simulink model "completo"  (R2022a)
settings: Solver=ode5  StartTime=0.0  StopTime=15  FixedStep=0.0001  RelTol=1e-3
InitFcn:
  | params_completo
values from neighbouring files (symbols this model uses):
  a = -1  /tau    (= -1000)    [params_completo.m]
  A_h = 0.40648    [params_completo.m]
  a_sat = (pi)/(2*(M_ij - L_ij))    (= 0.0314159265359)    [params_completo.m]
  alpha = 80    [params_completo.m]
  b = 1/tau    (= 1000)    [params_completo.m]
  beta1 = 0.0032    [params_completo.m]
  beta2 = 0.0035    [params_completo.m]
  beta3 = -0.0010    (= -0.001)    [params_completo.m]
  beta4 = -0.0003    [params_completo.m]
  beta5 = -0.0002    [params_completo.m]
  beta6 = 0.0004    [params_completo.m]
  freq = 2*pi/10    (= 0.628318530718)    [params_completo.m]
  k = 1.0773    [params_completo.m]
  k1 = 20    [params_completo.m]
  k1_o = 500    [params_completo.m]
  k2_o = 200    [params_completo.m]
  kx1 = 800    [params_completo.m]
  kx2 = 200    [params_completo.m]
  L_ij = 450    [params_completo.m]
  mu1 = 0.2    [params_completo.m]
  mu2 = 1.2    [params_completo.m]
  Phi_sum_abs = abs(beta1) + abs(beta2) + abs(beta3) +                abs(beta4) + abs(beta5) + abs(beta6)    [params_completo.m]
  Phi_sum_abs_ESTIMATED = Phi_sum_abs + 0.1 * Phi_sum_abs    [params_completo.m]
  q = 1    [params_completo.m]
settings Model: Creator=gerar  LastModifiedBy=CIO
settings SolverCC: AlgebraicLoopSolver=TrustRegion
settings DebuggingCC: UnconnectedInputMsg=warning  UnconnectedOutputMsg=warning  UnconnectedLineMsg=warning  SFMachineParentedDataDiag=warning
settings SFSimCC: CustomCodeUndefinedFunction=UseInterfaceOnly
settings RTWCC: DLArmComputeVersion=19.05

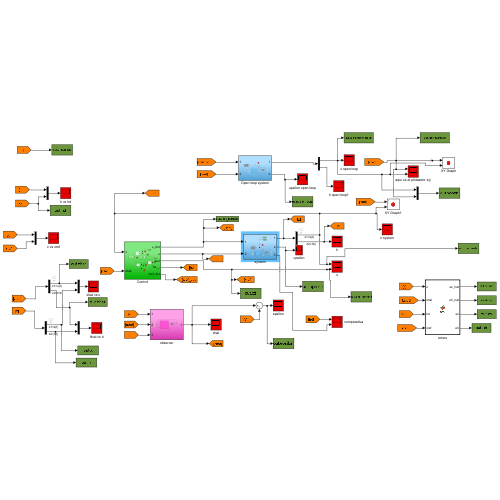
[thumbnail: Simulink's stored preview of the top-level diagram]
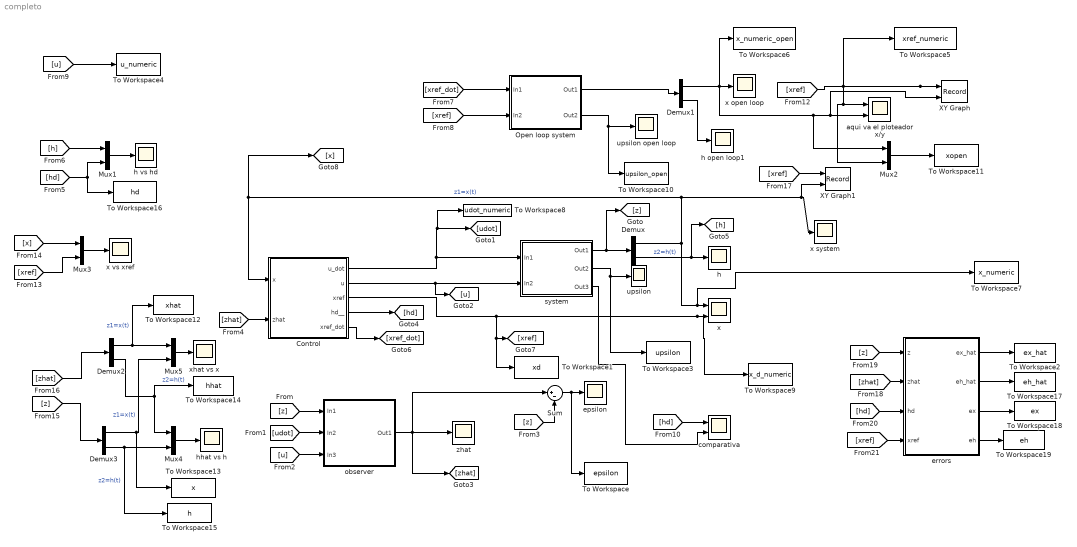
== system completo ==
  Control : Subsystem
  Demux{,1..3} (4 alike) : Demux  Outputs=2
  Mux{1..5} (5 alike) : Mux  Inputs=2
  Open loop system : Subsystem
  Sum : Sum  Inputs=|+-
  To Workspace : ToWorkspace  VariableName=epsilon  SaveFormat=Timeseries  SampleTime=-1
  To Workspace1 : ToWorkspace  VariableName=xd  SaveFormat=Timeseries  SampleTime=-1
  To Workspace10 : ToWorkspace  VariableName=upsilon_open  SaveFormat=Structure  SampleTime=-1
  To Workspace11 : ToWorkspace  VariableName=xopen  SaveFormat=Timeseries  SampleTime=-1
  To Workspace12 : ToWorkspace  VariableName=xhat  SaveFormat=Timeseries  SampleTime=-1
  To Workspace13 : ToWorkspace  VariableName=x  SaveFormat=Timeseries  SampleTime=-1
  To Workspace14 : ToWorkspace  VariableName=hhat  SaveFormat=Timeseries  SampleTime=-1
  To Workspace15 : ToWorkspace  VariableName=h  SaveFormat=Timeseries  SampleTime=-1
  To Workspace16 : ToWorkspace  VariableName=hd  SaveFormat=Timeseries  SampleTime=-1
  To Workspace17 : ToWorkspace  VariableName=eh_hat  SaveFormat=Timeseries  SampleTime=-1
  To Workspace18 : ToWorkspace  VariableName=ex  SaveFormat=Timeseries  SampleTime=-1
  To Workspace19 : ToWorkspace  VariableName=eh  SaveFormat=Timeseries  SampleTime=-1
  To Workspace2 : ToWorkspace  VariableName=ex_hat  SaveFormat=Timeseries  SampleTime=-1
  To Workspace3 : ToWorkspace  VariableName=upsilon  SaveFormat=Structure  SampleTime=-1
  To Workspace4 : ToWorkspace  VariableName=u_numeric  SaveFormat=Structure  SampleTime=-1
  To Workspace5 : ToWorkspace  VariableName=xref_numeric  SaveFormat=Structure  SampleTime=-1
  To Workspace6 : ToWorkspace  VariableName=x_numeric_open  SaveFormat=Structure  SampleTime=-1
  To Workspace7 : ToWorkspace  VariableName=x_numeric  SaveFormat=Structure  SampleTime=-1
  To Workspace8 : ToWorkspace  VariableName=udot_numeric  SaveFormat=Structure  SampleTime=-1
  To Workspace9 : ToWorkspace  VariableName=x_d_numeric  SaveFormat=Structure  SampleTime=-1
  XY Graph : Record  FileSettingsInternal="{\"entries\":[{\"content\":{\"excelSettings\":{\"content\":{},\"type\":\"Streamout.ExcelSettings\"}},\"type\":\"Streamout.FileSettingStorage\",\"uuid\":\"58948ec6-d345-4ba4-a5f9-32bad8470a1a\"}],\"packageUris\":[\"http://schema.mathworks.com/mf0/streamout_blocks/R2020a\"],\"version\":\"1.0\"}"  Layout=[1 1]  SignalsInternal="{\"entries\":[{\"content\":{\"signals\":[{\"content\":{\"blockPath\":[\"completo/XY Graph\"],\"channel\":[],\"dimensions\":[1],\"domain\":\"completo/XY Graph\",\"lineColor\":\"#a2142f\",\"plots\":[1],\"port\":1,\"sid\":[],\"signalID\":655,\"signalName\":\"From12\"},\"type\":\"RecordBlkView.Signal\",\"uuid\":\"ccf76168-5501-4964-b812-cd25957922a2\"},{\"content\":{\"blockPath\":[\"completo/XY Graph\"],\"channel\":[],\"dimensions\":[1],\"domain\":\"completo/XY Graph\",\"lineColor\":\"#139fff\",\"plots\":[1],\"port\":2,\"sid\":[],\"signalID\":658,\"signalName\":\"Demux1:1\"},\"type\":\"RecordBlkView.Signal\",\"uuid\":\"d05795eb-9c31-488d-9f29-71855a3ce2a9\"}]},\"type\":\"RecordBlkView.InputSignals\",\"uuid\":\"1ab41c32-35a5-46b4-97f6-ee8bfd3e0af7\"}],\"packageUris\":[\"http://schema.mathworks.com/mf0/streamout_blocks/R2020a\"],\"version\":\"1.0\"}"  VisualizationBindings="{\"xyplotplugin\":{\"info\":[{\"series\":[{\"bindingParametersList\":[{\"parameter\":\"X-Axis\",\"signalID\":655,\"signalName\":\"From12\"},{\"parameter\":\"Y-Axis\",\"signalID\":658,\"signalName\":\"Demux1:1\"}],\"seriesID\":39720}],\"subplotID\":1}]}}"  CompatibilityTag=XY
  XY Graph1 : Record  FileSettingsInternal="{\"entries\":[{\"content\":{\"excelSettings\":{\"content\":{},\"type\":\"Streamout.ExcelSettings\"}},\"type\":\"Streamout.FileSettingStorage\",\"uuid\":\"11f322b1-eef3-45be-a83d-5182385591cb\"}],\"packageUris\":[\"http://schema.mathworks.com/mf0/streamout_blocks/R2020a\"],\"version\":\"1.0\"}"  Layout=[1 1]  SignalsInternal="{\"entries\":[{\"content\":{\"signals\":[{\"content\":{\"blockPath\":[\"completo/XY Graph1\"],\"channel\":[],\"dimensions\":[1],\"domain\":\"completo/XY Graph1\",\"lineColor\":\"#a2142f\",\"plots\":[1],\"port\":1,\"sid\":[],\"signalID\":647,\"signalName\":\"From17\"},\"type\":\"RecordBlkView.Signal\",\"uuid\":\"a2b6a24d-7c32-44e8-9cda-e5b06c3ad770\"},{\"content\":{\"blockPath\":[\"completo/XY Graph1\"],\"channel\":[],\"dimensions\":[1],\"domain\":\"completo/XY Graph1\",\"lineColor\":\"#139fff\",\"plots\":[1],\"port\":2,\"sid\":[],\"signalID\":650,\"signalName\":\"z1=x(t)\"},\"type\":\"RecordBlkView.Signal\",\"uuid\":\"9a324e81-d58f-46a3-8cfa-1b0d0714c485\"}]},\"type\":\"RecordBlkView.InputSignals\",\"uuid\":\"4fdf8df6-887b-4fd8-83f4-ac5bb18b92d4\"}],\"packageUris\":[\"http://schema.mathworks.com/mf0/streamout_blocks/R2020a\"],\"version\":\"1.0\"}"  VisualizationBindings="{\"xyplotplugin\":{\"info\":[{\"series\":[{\"bindingParametersList\":[{\"parameter\":\"X-Axis\",\"signalID\":647,\"signalName\":\"From17\"},{\"parameter\":\"Y-Axis\",\"signalID\":650,\"signalName\":\"z1=x(t)\"}],\"seriesID\":20684}],\"subplotID\":1}]}}"  CompatibilityTag=XY
  aqui va el ploteador x/y : Scope  NumInputPorts=2
  comparativa : Scope  NumInputPorts=2
  epsilon : Scope
  errors : MATLAB Function  TreatAsAtomicUnit=on
  h : Scope
  h open loop1 : Scope
  h vs hd : Scope
  hhat vs h : Scope
  observer : Subsystem
  system : Subsystem
  upsilon : Scope
  upsilon open loop : Scope
  x : Scope  NumInputPorts=2
  x open loop : Scope
  x system : Scope
  x vs xref : Scope
  xhat vs x : Scope
  zhat : Scope
  wires:
  Control/1(u_dot) -> To Workspace8/1, [udot], system/1(In1)
  Control/2(u) -> system/2(In2), [u]
  Control/3(xref) -> To Workspace1/1, [xref], To Workspace9/1, x/2
  Demux/2 -> [h], h/1  "z2=h(t)"
  Demux/1 -> To Workspace7/1, x/1, XY Graph1/2, x system/1, [x], Control/1(x)  "z1=x(t)"
  system/1(Out1) -> Demux/1, [z]
  [z] -> observer/1(In1)
  observer/1(Out1) -> [zhat], Sum/1, zhat/1
  [udot] -> observer/2(In2)
  [u] -> observer/3(In3)
  [z] -> Sum/2
  Sum/1 -> To Workspace/1, epsilon/1
  [zhat] -> Control/2(zhat)
  system/2(Out2) -> To Workspace3/1, upsilon/1
  Control/4(hd__) -> [hd]
  [h] -> Mux1/1
  [hd] -> To Workspace16/1, Mux1/2
  Mux1/1 -> h vs hd/1
  Control/5(xref_dot) -> [xref_dot]
  [xref_dot] -> Open loop system/1(In1)
  [xref] -> Open loop system/2(In2)
  Open loop system/1(Out1) -> Demux1/1
  Open loop system/2(Out2) -> To Workspace10/1, upsilon open loop/1
  Demux1/2 -> h open loop1/1
  Demux1/1 -> To Workspace6/1, x open loop/1, XY Graph/2, aqui va el ploteador x/y/2, Mux2/1
  [u] -> To Workspace4/1
  system/3(Out3) -> comparativa/2
  [hd] -> comparativa/1
  [xref] -> XY Graph/1, To Workspace5/1, Mux2/2, aqui va el ploteador x/y/1
  Mux2/1 -> To Workspace11/1
  [xref] -> Mux3/2
  [x] -> Mux3/1
  Mux3/1 -> x vs xref/1
  [xref] -> XY Graph1/1
  [zhat] -> Demux2/1
  [z] -> Demux3/1
  Demux2/1 -> To Workspace12/1, Mux5/1  "z1=x(t)"
  Demux3/1 -> To Workspace13/1, Mux5/2  "z1=x(t)"
  Mux5/1 -> xhat vs x/1
  Demux2/2 -> To Workspace14/1, Mux4/1  "z2=h(t)"
  Demux3/2 -> To Workspace15/1, Mux4/2  "z2=h(t)"
  Mux4/1 -> hhat vs h/1
  [zhat] -> errors/2(zhat)
  [z] -> errors/1(z)
  [hd] -> errors/3(hd)
  [xref] -> errors/4(xref)
  errors/1(ex_hat) -> To Workspace2/1
  errors/2(eh_hat) -> To Workspace17/1
  errors/3(ex) -> To Workspace18/1
  errors/4(eh) -> To Workspace19/1

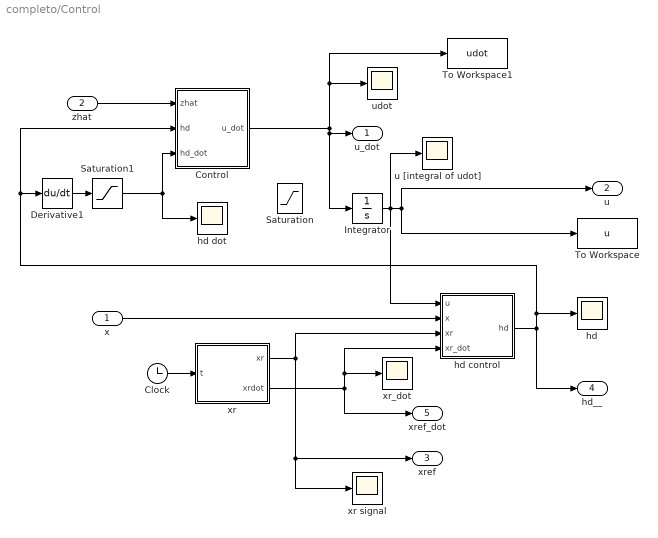
== system completo/Control ==
  x : Inport
  zhat : Inport  Port=2
  Clock : Clock
  Control : MATLAB Function  TreatAsAtomicUnit=on
  Derivative1 : Derivative
  Integrator : Integrator
  Saturation : Saturate  UpperLimit=100  LowerLimit=-100
  Saturation1 : Saturate  UpperLimit=40  LowerLimit=-40
  To Workspace : ToWorkspace  VariableName=u  SaveFormat=Timeseries  SampleTime=-1
  To Workspace1 : ToWorkspace  VariableName=udot  SaveFormat=Timeseries  SampleTime=-1
  hd : Scope
  hd control : MATLAB Function  TreatAsAtomicUnit=on
  hd dot : Scope
  u [integral of udot] : Scope
  udot : Scope
  xr : MATLAB Function  TreatAsAtomicUnit=on
  xr signal : Scope
  xr_dot : Scope
  u_dot : Outport  VectorParamsAs1DForOutWhenUnconnected=off
  u : Outport  Port=2  VectorParamsAs1DForOutWhenUnconnected=off
  xref : Outport  Port=3  VectorParamsAs1DForOutWhenUnconnected=off
  hd__ : Outport  Port=4  VectorParamsAs1DForOutWhenUnconnected=off
  xref_dot : Outport  Port=5  VectorParamsAs1DForOutWhenUnconnected=off
  wires:
  Integrator/1 -> hd control/1(u), To Workspace/1, u/1, u [integral of udot]/1
  x/1 -> hd control/2(x)
  Clock/1 -> xr/1(t)
  xr/1(xr) -> xr signal/1, xref/1, hd control/3(xr)
  zhat/1 -> Control/1(zhat)
  xr/2(xrdot) -> xref_dot/1, hd control/4(xr_dot), xr_dot/1
  Derivative1/1 -> Saturation1/1
  Saturation1/1 -> hd dot/1, Control/3(hd_dot)
  hd control/1(hd) -> hd/1, Control/2(hd), Derivative1/1, hd__/1
  Control/1(u_dot) -> Integrator/1, u_dot/1, udot/1, To Workspace1/1

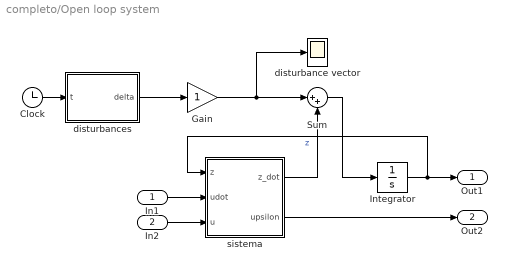
== system completo/Open loop system ==
  In1 : Inport
  In2 : Inport  Port=2
  Clock : Clock
  Gain : Gain
  Integrator : Integrator  InitialCondition=[3;-2]
  Sum : Sum  Inputs=|++
  disturbance vector : Scope
  disturbances : MATLAB Function  TreatAsAtomicUnit=on
  sistema : MATLAB Function  TreatAsAtomicUnit=on
  Out1 : Outport  VectorParamsAs1DForOutWhenUnconnected=off
  Out2 : Outport  Port=2  VectorParamsAs1DForOutWhenUnconnected=off
  wires:
  Integrator/1 -> Out1/1, sistema/1(z)  "z"
  In1/1 -> sistema/2(udot)
  In2/1 -> sistema/3(u)
  sistema/2(upsilon) -> Out2/1
  Clock/1 -> disturbances/1(t)
  sistema/1(z_dot) -> Sum/2
  disturbances/1(delta) -> Gain/1
  Sum/1 -> Integrator/1
  Gain/1 -> Sum/1, disturbance vector/1

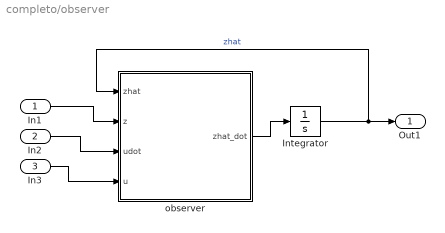
== system completo/observer ==
  In1 : Inport
  In2 : Inport  Port=2
  In3 : Inport  Port=3
  Integrator : Integrator  InitialCondition=[0;0]
  observer : MATLAB Function  TreatAsAtomicUnit=on
  Out1 : Outport  VectorParamsAs1DForOutWhenUnconnected=off
  wires:
  observer/1(zhat_dot) -> Integrator/1
  Integrator/1 -> observer/1(zhat), Out1/1  "zhat"
  In1/1 -> observer/2(z)
  In2/1 -> observer/3(udot)
  In3/1 -> observer/4(u)

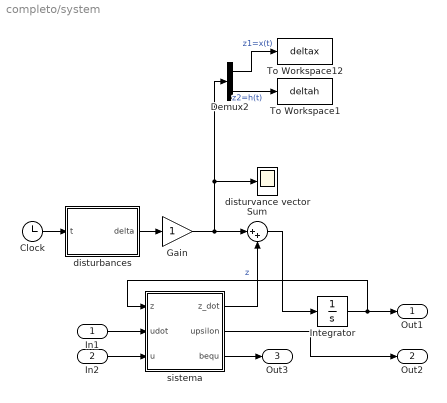
== system completo/system ==
  In1 : Inport
  In2 : Inport  Port=2
  Clock : Clock
  Demux2 : Demux  Outputs=2
  Gain : Gain
  Integrator : Integrator  InitialCondition=[3;-2]
  Sum : Sum  Inputs=|++
  To Workspace1 : ToWorkspace  VariableName=deltah  SaveFormat=Timeseries  SampleTime=-1
  To Workspace12 : ToWorkspace  VariableName=deltax  SaveFormat=Timeseries  SampleTime=-1
  disturbances : MATLAB Function  TreatAsAtomicUnit=on
  disturvance vector : Scope
  sistema : MATLAB Function  TreatAsAtomicUnit=on
  Out1 : Outport  VectorParamsAs1DForOutWhenUnconnected=off
  Out2 : Outport  Port=2  VectorParamsAs1DForOutWhenUnconnected=off
  Out3 : Outport  Port=3  VectorParamsAs1DForOutWhenUnconnected=off
  wires:
  Integrator/1 -> Out1/1, sistema/1(z)  "z"
  In1/1 -> sistema/2(udot)
  In2/1 -> sistema/3(u)
  sistema/2(upsilon) -> Out2/1
  Clock/1 -> disturbances/1(t)
  sistema/1(z_dot) -> Sum/2
  disturbances/1(delta) -> Gain/1
  Sum/1 -> Integrator/1
  sistema/3(bequ) -> Out3/1
  Gain/1 -> Demux2/1, disturvance vector/1, Sum/1
  Demux2/1 -> To Workspace12/1  "z1=x(t)"
  Demux2/2 -> To Workspace1/1  "z2=h(t)"

== matlab function completo/Open loop system/disturbances ==
  data: t input; delta output
function delta = dist(t)

delta_x = -3 - 10*cos(0.2*t+10);
delta_h = 8*sin(t); 

delta = [delta_x ; delta_h];

== matlab function completo/Open loop system/sistema ==
  data: z input; udot input; u input; z_dot output; k parameter; a parameter; b parameter; upsilon output; beta1 parameter; beta2 parameter; beta3 parameter; beta4 parameter; beta5 parameter; beta6 parameter; A_h parameter
function [z_dot, upsilon] = sys(z, udot, u, k, a, b, beta1, beta2, beta3, beta4, beta5, beta6, A_h)

    x = z(1,1);
    h = z(2,1);

    Phi = beta1*sign( udot*h ) + beta2*sign( udot*u ) + ...
          beta3*sign( u*h )    + beta4*sign( udot )   + ...
          beta5*sign( h )      + beta6*sign( u );

    %============================ System model ============================
    z_dot = [ a*x + b*k*u - b*h    ;    
            udot*( A_h - abs(h)*Phi ) ];

    upsilon = k*u - h;
    bequ = b*k*u;

== matlab function completo/errors ==
  data: z input; zhat input; hd input; ex_hat output; xref input; eh_hat output; ex output; eh output
function [ex_hat, eh_hat, ex, eh] = fcn(z, zhat, hd, xref)

x = z(1,1);
h = z(2,1);

xhat = zhat(1,1);
hhat = zhat(2,1);



%%%
ex_hat = xhat - x;
eh_hat = hhat - h;

ex = x - xref;
eh = h - hd;

== matlab function completo/Control/Control ==
  data: zhat input; hd input; hd_dot input; u_dot output; k1 parameter; A_h parameter; Phi_sum_abs parameter; Phi_sum_abs_ESTIMATED parameter
function u_dot = fcn(zhat, hd, hd_dot, k1, A_h, Phi_sum_abs, Phi_sum_abs_ESTIMATED)

eh = zhat(2,1) - hd;  %error with estimated states

%%%%%%%%%%%%%%%%%%% CO N T R O L %%%%%%%%%%%%%%%%%%%%%%%%%%%%%%%%%

u_dot = ( - k1 * sign(eh) + hd_dot )/( A_h - (Phi_sum_abs)*abs(eh + hd) ) ;

== matlab function completo/system/disturbances ==
  data: t input; delta output
function delta = dist(t)

delta_x = -3 - 10*cos(0.2*t+10);
delta_h = 8*sin(t); 

delta = [delta_x ; delta_h];

== matlab function completo/observer/observer ==
  data: zhat input; z input; udot input; u input; zhat_dot output; A_h parameter; k parameter; a parameter; b parameter; Phi_sum_abs_ESTIMATED parameter; k1_o parameter; k2_o parameter; mu1 parameter; mu2 parameter; q parameter
function zhat_dot = obs(zhat, z, udot, u, A_h, k, a, b, Phi_sum_abs_ESTIMATED, k1_o, k2_o, mu1, mu2, q)

x = z(1,1);
xhat = zhat(1,1);
hhat = zhat(2,1);


    gx = [ a*xhat + b*k*u - b*hhat                        ; %    gx = [ a*xhat + b*k*u                          ; 
          ( udot ) * ( A_h - abs(hhat)*Phi_sum_abs_ESTIMATED ) ] ;


%%%%%%%%%%%%%%%%%%%%%%%% o b s e r v e r %%%%%%%%%%%%%%%%%%%%%%%%%%%%%%%%%%
%error
e1 = xhat - x; 

%functions
phi1 = mu1*abs(e1)^(1/2)*sign(e1) + mu2 * abs(e1)^q * sign(e1)      ; 
phi2 = ( (mu1/2)*abs(e1)^(-1/2) + mu2*q*abs(e1)^(q-1) ) * ( phi1 ); 
correction_term = [- k1_o * phi1;
                   - k2_o * phi2];

zhat_dot =  gx -  correction_term;

== matlab function completo/Control/hd control ==
  data: u input; x input; xr input; xr_dot input; hd output; k parameter; a parameter; b parameter; L_ij parameter; kx1 parameter; kx2 parameter; a_sat parameter
function hd = fcn(u, x, xr, xr_dot, k, a, b, L_ij, kx1, kx2, a_sat)

ex = x - xr;

%%%%%%%%%%%%%%%%%%%%%%%% C O N T R O L  %%%%%%%%%%%%%%%%%%%%%%%%%%%

s = kx1*ex; % kx1

if s > L_ij
    sigma = tanh(a_sat*(s - L_ij))/(a_sat) + L_ij;
elseif abs(s) <= L_ij
    sigma = s;
elseif s < (-L_ij)
    sigma = tanh(a_sat*(s + L_ij))/(a_sat) - L_ij;
else
    sigma = 0;
end
    
hd = (1/b) * ( - sigma - kx2*sign(ex) + a*(ex + xr) + b*k*u - xr_dot );

== matlab function completo/Control/xr ==
  data: t input; xr output; alpha parameter; xrdot output; freq parameter
function [xr, xrdot] = fcn(t, alpha, freq)

xr = alpha*sin(freq*t);
xrdot = freq*alpha*cos(freq*t);

== matlab function completo/system/sistema ==
  data: z input; udot input; u input; z_dot output; A_h parameter; k parameter; a parameter; b parameter; upsilon output; bequ output; beta1 parameter; beta2 parameter; beta3 parameter; beta4 parameter; beta5 parameter; beta6 parameter
function [z_dot, upsilon, bequ] = sys(z, udot, u, A_h, k, a, b, beta1, beta2, beta3, beta4, beta5, beta6)

    x = z(1,1);
    h = z(2,1);

    Phi = beta1*sign( udot*h ) + beta2*sign( udot*u ) + ...
          beta3*sign( u*h )    + beta4*sign( udot )   + ...
          beta5*sign( h )      + beta6*sign( u );

    %============================ System model ============================
    % System:
    z_dot = [ a*x + b*k*u - b*h    ;    
            udot*( A_h - abs(h)*Phi ) ];

    upsilon = k*u - h;
    bequ = b*k*u;
